simulink model "Program_3_China_Simple_SIR_R2018a"  (R2018a)
settings: Solver=VariableStepAuto  StartTime=0.0  StopTime=90  RelTol=1e-9  AbsTol=1e-9
undefined symbols (not defined in the file): beta, C0, gamma, I0, N, R0
libraries: simulink x1
settings Model: OrderedModelArguments=off  Creator=ismae  LastModifiedBy=ismae
settings SolverCC: SolverResetMethod=Robust
settings DataIOCC: ReturnWorkspaceOutputs=on
settings SFSimCC: SimUseLocalCustomCode=on
settings RTWCC: RTWUseLocalCustomCode=on

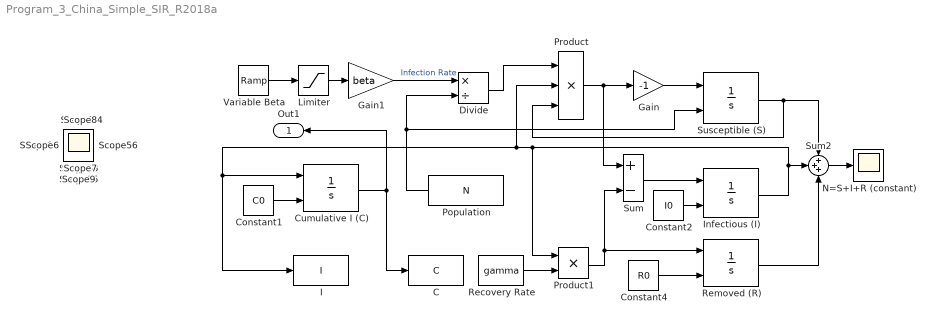
== system Program_3_China_Simple_SIR_R2018a ==
  C : ToWorkspace  VariableName=C  SampleTime=1
      settings: Save2DSignal=2-D array (concatenate along first dimension)
  Constant1 : Constant  Value=C0
  Constant2 : Constant  Value=I0
  Constant4 : Constant  Value=R0
  Cumulative I (C) : Integrator  InitialConditionSource=external
  Divide : Product  Inputs=*/
  Gain : Gain  Gain=-1
  Gain1 : Gain  Gain=beta
  I : ToWorkspace  VariableName=I  SampleTime=1
      settings: Save2DSignal=2-D array (concatenate along first dimension)
  Infectious (I) : Integrator  InitialConditionSource=external
  Limiter : Saturate  UpperLimit=2  LowerLimit=0.3
  N=S+I+R (constant) : Scope
  Population : Constant  Value=N
  Product : Product  Inputs=3
  Product1 : Product
  Recovery Rate : Constant  Value=gamma
  Removed (R) : Integrator  InitialConditionSource=external
  Sum : Sum  Inputs=+-
  Sum2 : Sum  Inputs=+++
  "Susceptible (S) " : Integrator  InitialConditionSource=external  InitialCondition=10000
  Variable Beta : simulink/Sources/Ramp  slope=-0.00268  start=0  InitialOutput=0.7  VectorParams1D=off
  Out1 : Outport
  Scope{,1..17} (18 alike) : Scope
  wires:
  Limiter/1 -> Gain1/1
  Gain/1 -> "Susceptible (S) "/1
  Population/1 -> Divide/2, "Susceptible (S) "/2
  Removed (R)/1 -> Sum2/3
  Variable Beta/1 -> Limiter/1
  Gain1/1 -> Divide/1  "Infection Rate"
  Infectious (I)/1 -> I/1, Cumulative I (C)/1, Product/2, Product1/1, Sum2/2
  Sum2/1 -> N=S+I+R (constant)/1
  Constant2/1 -> Infectious (I)/2
  Cumulative I (C)/1 -> Out1/1, C/1
  Constant4/1 -> Removed (R)/2
  Product/1 -> Sum/1, Gain/1
  Sum/1 -> Infectious (I)/1
  "Susceptible (S) "/1 -> Product/3, Sum2/1
  Recovery Rate/1 -> Product1/2
  Divide/1 -> Product/1
  Product1/1 -> Sum/2, Removed (R)/1
  Constant1/1 -> Cumulative I (C)/2
